simulink model "scheme"  (R2025b)
settings: Solver=VariableStepAuto  StartTime=0.0  StopTime=20.0  RelTol=1e-3
settings Model: Creator=Teacher  LastModifiedBy=lucag
settings SolverCC: AlgebraicLoopSolver=TrustRegion
settings DebuggingCC: UnconnectedInputMsg=warning  UnconnectedOutputMsg=warning  UnconnectedLineMsg=warning
settings ModelReferenceCC: EnableRefExpFcnMdlSchedulingChecks=on
settings RTWCC: GPUComputeCapability=3.5

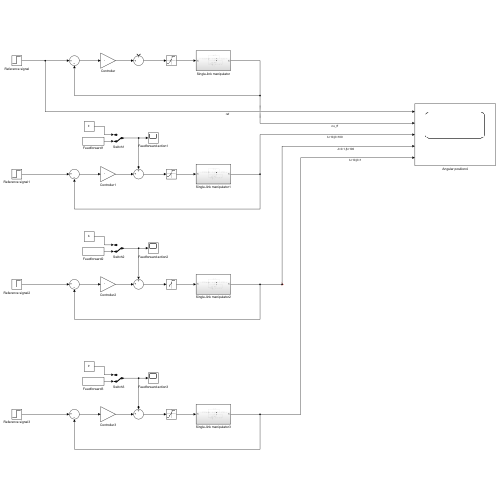
[thumbnail: Simulink's stored preview of the top-level diagram]
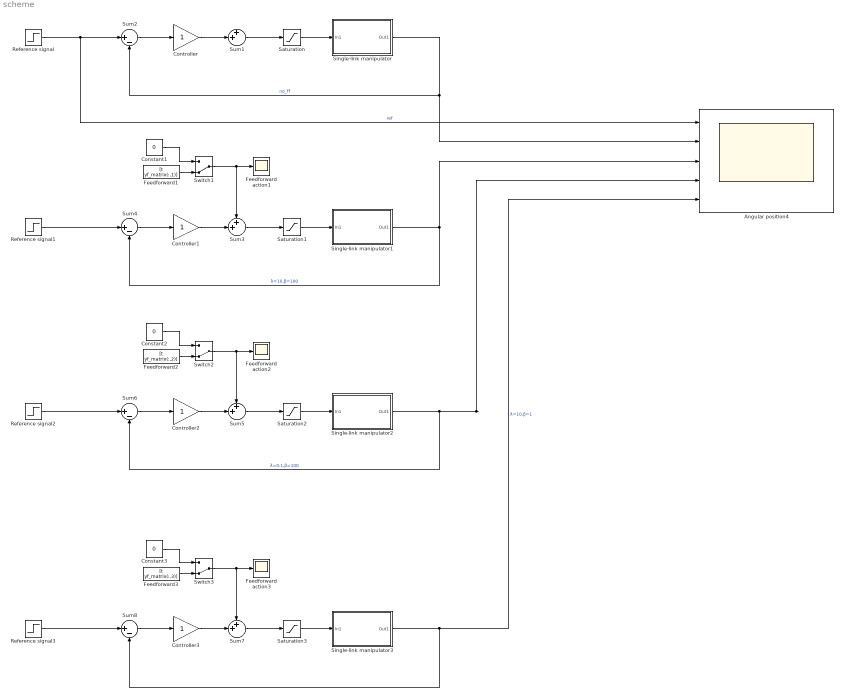
== system scheme ==
  Angular position4 : Scope  NumInputPorts=5
      settings: ActiveDisplayYMinimum=-1.1719015514764557  ActiveDisplayYMaximum=11.114346067571162  DataLoggingVariableName=ScopeData7
  Constant1 : Constant  Value=0
  Constant2 : Constant  Value=0
  Constant3 : Constant  Value=0
  Controller{,1..3} (4 alike) : Gain
  Feedforward action1 : Scope
      settings: ActiveDisplayYMinimum=-1.22324  ActiveDisplayYMaximum=6.26117  DataLoggingVariableName=ScopeData2
  Feedforward action2 : Scope
      settings: ActiveDisplayYMinimum=-1.22324  ActiveDisplayYMaximum=6.26117  DataLoggingVariableName=ScopeData4
  Feedforward action3 : Scope
      settings: ActiveDisplayYMinimum=-1.22324  ActiveDisplayYMaximum=6.26117  DataLoggingVariableName=ScopeData6
  Feedforward1 : FromWorkspace  VariableName=[t yf_matrix(:,1)]
  Feedforward2 : FromWorkspace  VariableName=[t yf_matrix(:,2)]
  Feedforward3 : FromWorkspace  VariableName=[t yf_matrix(:,3)]
  Reference signal{,1..3} (4 alike) : Step  After=10  SampleTime=0
  Saturation{,1..3} (4 alike) : Saturate  UpperLimit=10  LowerLimit=-10
  Single-link manipulator : Subsystem
  Single-link manipulator1 : Subsystem
  Single-link manipulator2 : Subsystem
  Single-link manipulator3 : Subsystem
  Sum{1,3,5,7} (4 alike) : Sum  Inputs=++|
  Sum{2,4,6,8} (4 alike) : Sum  Inputs=|+-
  Switch1 : ManualSwitch  CurrentSetting=0
  Switch2 : ManualSwitch  CurrentSetting=0
  Switch3 : ManualSwitch  CurrentSetting=0
  wires:
  Sum2/1 -> Controller/1
  Controller/1 -> Sum1/2
  Sum1/1 -> Saturation/1
  Single-link manipulator/1(Out1) -> Angular position4/2, Sum2/2  "no_ff"
  Saturation/1 -> Single-link manipulator/1(In1)
  Feedforward1/1 -> Switch1/2
  Reference signal1/1 -> Sum4/1
  Sum4/1 -> Controller1/1
  Saturation1/1 -> Single-link manipulator1/1(In1)
  Controller1/1 -> Sum3/2
  Constant1/1 -> Switch1/1
  Switch1/1 -> Feedforward action1/1, Sum3/1
  Sum3/1 -> Saturation1/1
  Sum5/1 -> Saturation2/1
  Saturation2/1 -> Single-link manipulator2/1(In1)
  Constant2/1 -> Switch2/1
  Controller2/1 -> Sum5/2
  Sum6/1 -> Controller2/1
  Reference signal2/1 -> Sum6/1
  Feedforward2/1 -> Switch2/2
  Switch2/1 -> Feedforward action2/1, Sum5/1
  Switch3/1 -> Feedforward action3/1, Sum7/1
  Sum8/1 -> Controller3/1
  Feedforward3/1 -> Switch3/2
  Controller3/1 -> Sum7/2
  Saturation3/1 -> Single-link manipulator3/1(In1)
  Reference signal3/1 -> Sum8/1
  Constant3/1 -> Switch3/1
  Sum7/1 -> Saturation3/1
  Single-link manipulator3/1(Out1) -> Angular position4/5, Sum8/2  "λ=10,β=1"
  Single-link manipulator2/1(Out1) -> Sum6/2, Angular position4/4  "λ=0.1,β=100"
  Reference signal/1 -> Angular position4/1, Sum2/1  "ref"
  Single-link manipulator1/1(Out1) -> Angular position4/3, Sum4/2  "λ=10,β=100"

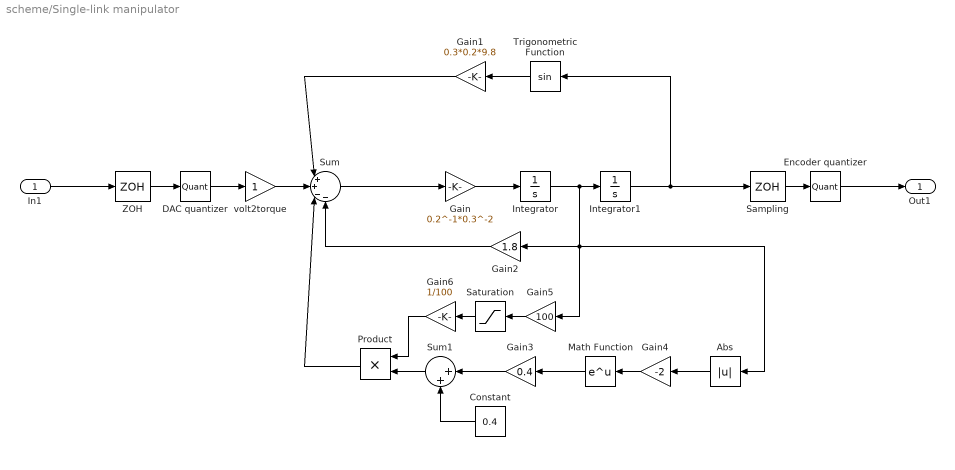
== system scheme/Single-link manipulator ==
  In1 : Inport
  Abs : Abs  SaturateOnIntegerOverflow=off
  Constant : Constant  Value=0.4
  DAC quantizer : Quantizer  QuantizationInterval=10/2^13
  Encoder quantizer : Quantizer  QuantizationInterval=2*pi/3000
  Gain : Gain  Gain=0.2^-1*0.3^-2
  Gain1 : Gain  Gain=0.3*0.2*9.8
  Gain2 : Gain  Gain=1.8
  Gain3 : Gain  Gain=0.4
  Gain4 : Gain  Gain=-2
  Gain5 : Gain  Gain=100
  Gain6 : Gain  Gain=1/100
  Integrator : Integrator
  Integrator1 : Integrator
  Math Function : Math
  Product : Product
  Sampling : ZeroOrderHold  SampleTime=0.001
  Saturation : Saturate  UpperLimit=1  LowerLimit=-1
  Sum : Sum  Inputs=|++--
  Sum1 : Sum  Inputs=|++
  Trigonometric Function : Trigonometry
  ZOH : ZeroOrderHold  SampleTime=0.001
  volt2torque : Gain
  Out1 : Outport
  wires:
  Gain/1 -> Integrator/1
  Gain3/1 -> Sum1/1
  Sum1/1 -> Product/2
  Gain6/1 -> Product/1
  Gain5/1 -> Saturation/1
  Gain2/1 -> Sum/4
  Gain1/1 -> Sum/1
  Integrator1/1 -> Sampling/1, Trigonometric Function/1
  Saturation/1 -> Gain6/1
  Trigonometric Function/1 -> Gain1/1
  Product/1 -> Sum/3
  Sum/1 -> Gain/1
  Constant/1 -> Sum1/2
  Integrator/1 -> Gain5/1, Abs/1, Gain2/1, Integrator1/1
  Abs/1 -> Gain4/1
  Gain4/1 -> Math Function/1
  Math Function/1 -> Gain3/1
  Sampling/1 -> Encoder quantizer/1
  Encoder quantizer/1 -> Out1/1
  ZOH/1 -> DAC quantizer/1
  DAC quantizer/1 -> volt2torque/1
  volt2torque/1 -> Sum/2
  In1/1 -> ZOH/1

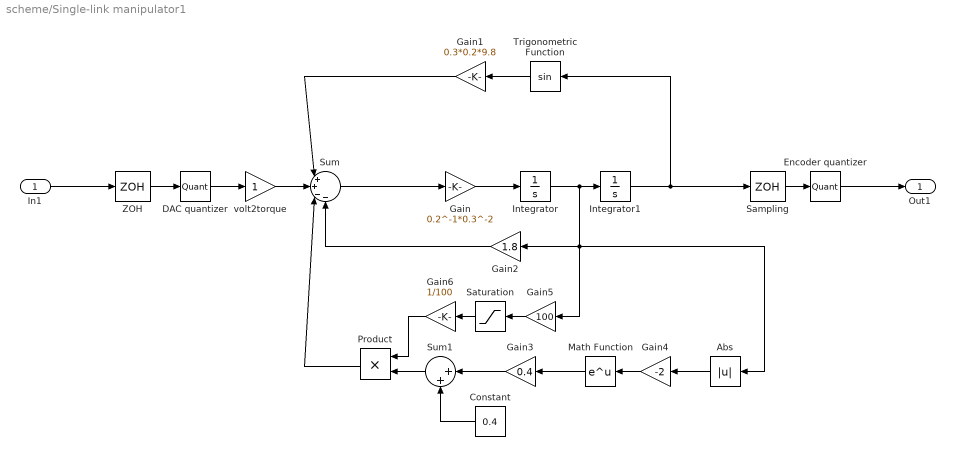
== system scheme/Single-link manipulator1 ==
  In1 : Inport
  Abs : Abs  SaturateOnIntegerOverflow=off
  Constant : Constant  Value=0.4
  DAC quantizer : Quantizer  QuantizationInterval=10/2^13
  Encoder quantizer : Quantizer  QuantizationInterval=2*pi/3000
  Gain : Gain  Gain=0.2^-1*0.3^-2
  Gain1 : Gain  Gain=0.3*0.2*9.8
  Gain2 : Gain  Gain=1.8
  Gain3 : Gain  Gain=0.4
  Gain4 : Gain  Gain=-2
  Gain5 : Gain  Gain=100
  Gain6 : Gain  Gain=1/100
  Integrator : Integrator
  Integrator1 : Integrator
  Math Function : Math
  Product : Product
  Sampling : ZeroOrderHold  SampleTime=0.001
  Saturation : Saturate  UpperLimit=1  LowerLimit=-1
  Sum : Sum  Inputs=|++--
  Sum1 : Sum  Inputs=|++
  Trigonometric Function : Trigonometry
  ZOH : ZeroOrderHold  SampleTime=0.001
  volt2torque : Gain
  Out1 : Outport
  wires:
  Gain/1 -> Integrator/1
  Gain3/1 -> Sum1/1
  Sum1/1 -> Product/2
  Gain6/1 -> Product/1
  Gain5/1 -> Saturation/1
  Gain2/1 -> Sum/4
  Gain1/1 -> Sum/1
  Integrator1/1 -> Sampling/1, Trigonometric Function/1
  Saturation/1 -> Gain6/1
  Trigonometric Function/1 -> Gain1/1
  Product/1 -> Sum/3
  Sum/1 -> Gain/1
  Constant/1 -> Sum1/2
  Integrator/1 -> Gain5/1, Abs/1, Gain2/1, Integrator1/1
  Abs/1 -> Gain4/1
  Gain4/1 -> Math Function/1
  Math Function/1 -> Gain3/1
  Sampling/1 -> Encoder quantizer/1
  Encoder quantizer/1 -> Out1/1
  ZOH/1 -> DAC quantizer/1
  DAC quantizer/1 -> volt2torque/1
  volt2torque/1 -> Sum/2
  In1/1 -> ZOH/1

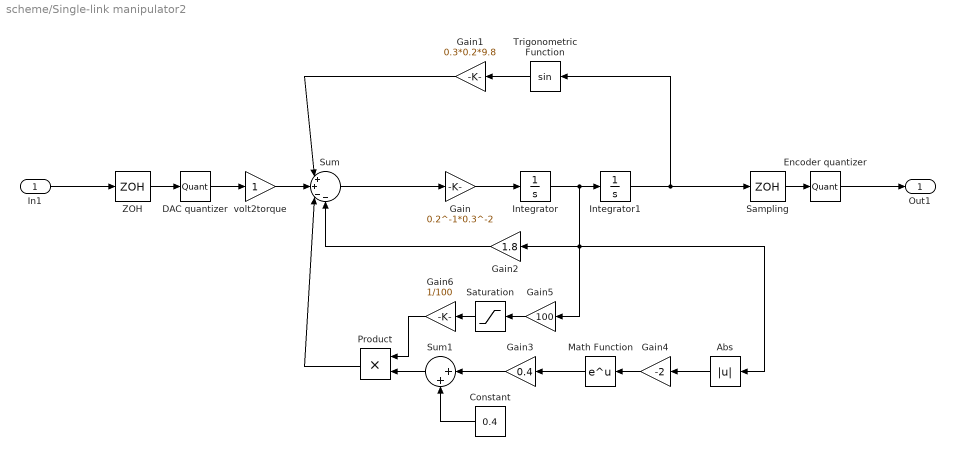
== system scheme/Single-link manipulator2 ==
  In1 : Inport
  Abs : Abs  SaturateOnIntegerOverflow=off
  Constant : Constant  Value=0.4
  DAC quantizer : Quantizer  QuantizationInterval=10/2^13
  Encoder quantizer : Quantizer  QuantizationInterval=2*pi/3000
  Gain : Gain  Gain=0.2^-1*0.3^-2
  Gain1 : Gain  Gain=0.3*0.2*9.8
  Gain2 : Gain  Gain=1.8
  Gain3 : Gain  Gain=0.4
  Gain4 : Gain  Gain=-2
  Gain5 : Gain  Gain=100
  Gain6 : Gain  Gain=1/100
  Integrator : Integrator
  Integrator1 : Integrator
  Math Function : Math
  Product : Product
  Sampling : ZeroOrderHold  SampleTime=0.001
  Saturation : Saturate  UpperLimit=1  LowerLimit=-1
  Sum : Sum  Inputs=|++--
  Sum1 : Sum  Inputs=|++
  Trigonometric Function : Trigonometry
  ZOH : ZeroOrderHold  SampleTime=0.001
  volt2torque : Gain
  Out1 : Outport
  wires:
  Gain/1 -> Integrator/1
  Gain3/1 -> Sum1/1
  Sum1/1 -> Product/2
  Gain6/1 -> Product/1
  Gain5/1 -> Saturation/1
  Gain2/1 -> Sum/4
  Gain1/1 -> Sum/1
  Integrator1/1 -> Sampling/1, Trigonometric Function/1
  Saturation/1 -> Gain6/1
  Trigonometric Function/1 -> Gain1/1
  Product/1 -> Sum/3
  Sum/1 -> Gain/1
  Constant/1 -> Sum1/2
  Integrator/1 -> Gain5/1, Abs/1, Gain2/1, Integrator1/1
  Abs/1 -> Gain4/1
  Gain4/1 -> Math Function/1
  Math Function/1 -> Gain3/1
  Sampling/1 -> Encoder quantizer/1
  Encoder quantizer/1 -> Out1/1
  ZOH/1 -> DAC quantizer/1
  DAC quantizer/1 -> volt2torque/1
  volt2torque/1 -> Sum/2
  In1/1 -> ZOH/1

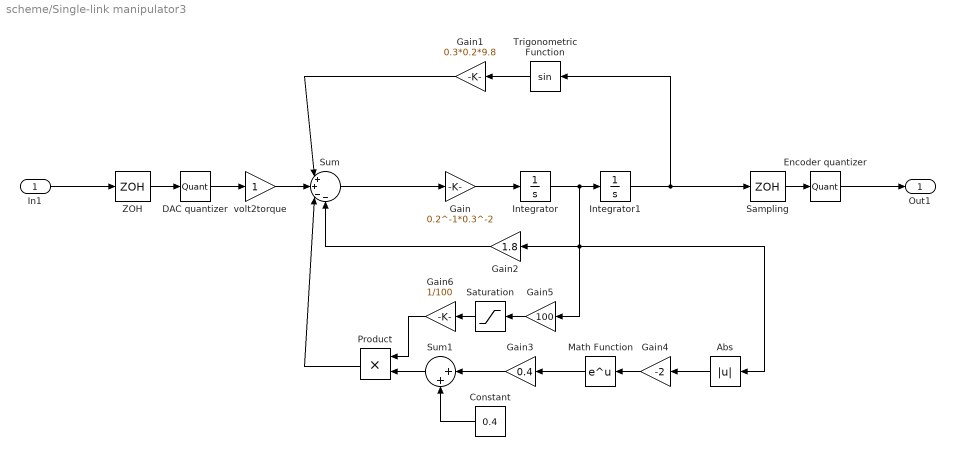
== system scheme/Single-link manipulator3 ==
  In1 : Inport
  Abs : Abs  SaturateOnIntegerOverflow=off
  Constant : Constant  Value=0.4
  DAC quantizer : Quantizer  QuantizationInterval=10/2^13
  Encoder quantizer : Quantizer  QuantizationInterval=2*pi/3000
  Gain : Gain  Gain=0.2^-1*0.3^-2
  Gain1 : Gain  Gain=0.3*0.2*9.8
  Gain2 : Gain  Gain=1.8
  Gain3 : Gain  Gain=0.4
  Gain4 : Gain  Gain=-2
  Gain5 : Gain  Gain=100
  Gain6 : Gain  Gain=1/100
  Integrator : Integrator
  Integrator1 : Integrator
  Math Function : Math
  Product : Product
  Sampling : ZeroOrderHold  SampleTime=0.001
  Saturation : Saturate  UpperLimit=1  LowerLimit=-1
  Sum : Sum  Inputs=|++--
  Sum1 : Sum  Inputs=|++
  Trigonometric Function : Trigonometry
  ZOH : ZeroOrderHold  SampleTime=0.001
  volt2torque : Gain
  Out1 : Outport
  wires:
  Gain/1 -> Integrator/1
  Gain3/1 -> Sum1/1
  Sum1/1 -> Product/2
  Gain6/1 -> Product/1
  Gain5/1 -> Saturation/1
  Gain2/1 -> Sum/4
  Gain1/1 -> Sum/1
  Integrator1/1 -> Sampling/1, Trigonometric Function/1
  Saturation/1 -> Gain6/1
  Trigonometric Function/1 -> Gain1/1
  Product/1 -> Sum/3
  Sum/1 -> Gain/1
  Constant/1 -> Sum1/2
  Integrator/1 -> Gain5/1, Abs/1, Gain2/1, Integrator1/1
  Abs/1 -> Gain4/1
  Gain4/1 -> Math Function/1
  Math Function/1 -> Gain3/1
  Sampling/1 -> Encoder quantizer/1
  Encoder quantizer/1 -> Out1/1
  ZOH/1 -> DAC quantizer/1
  DAC quantizer/1 -> volt2torque/1
  volt2torque/1 -> Sum/2
  In1/1 -> ZOH/1
